simulink model "ctrl_joy"  (R2020b)
settings: Solver=FixedStepAuto  StartTime=0.0  StopTime=Inf  FixedStep=0.01  RelTol=1e-3  EnableMultiTasking=on
model workspace (MAT data in the model file):
  SL_ROS_VariableLengthArrays_MaxSizes.CommonInfo.ArrayTruncateAction = 'EmitWarning'
  SL_ROS_VariableLengthArrays_MaxSizes.MsgTypeMap = containers.Map
  SL_ROS_VariableLengthArrays_MaxSizes.MsgTypeMap.serialization.keys = {'std_msgs/MultiArrayDimension', 'std_msgs/MultiArrayLayout'}
  SL_ROS_VariableLengthArrays_MaxSizes.MsgTypeMap.serialization.values{1}.PropertyName = 'Label'
  SL_ROS_VariableLengthArrays_MaxSizes.MsgTypeMap.serialization.values{1}.DataType = 'uint8'
  SL_ROS_VariableLengthArrays_MaxSizes.MsgTypeMap.serialization.values{1}.MaxLength = 2
  SL_ROS_VariableLengthArrays_MaxSizes.MsgTypeMap.serialization.values{2}.PropertyName = 'Dim'
  SL_ROS_VariableLengthArrays_MaxSizes.MsgTypeMap.serialization.values{2}.DataType = 'std_msgs/MultiArrayDimension'
  SL_ROS_VariableLengthArrays_MaxSizes.MsgTypeMap.serialization.values{2}.MaxLength = 1
  SL_ROS_VariableLengthArrays_MaxSizes.MsgTypeMap.serialization.uniformity = 0
  SL_ROS_VariableLengthArrays_MaxSizes.MsgTypeMap.serialization.keyType = 'char'
  SL_ROS_VariableLengthArrays_MaxSizes.MsgTypeMap.serialization.valueType = 'any'
undefined symbols (not defined in the file): Data, Data_SL_Info, Layout
libraries: robotlib x8
settings Model: SimulationMode=external  ExtModeEnableFloating=off  Creator=erlendbasso  LastModifiedBy=erlendbasso
settings SolverCC: PositivePriorityOrder=on
settings OptimizationCC: EnhancedBackFolding=on  PassReuseOutputArgsAs=Individual arguments  ZeroExternalMemoryAtStartup=off  ZeroInternalMemoryAtStartup=off  MaxStackSize=64  OptimizeBlockOrder=speed  DifferentSizesBufferReuse=on  OptimizationCustomize=off  EfficientTunableParamExpr=on
settings DebuggingCC: ParameterTunabilityLossMsg=error
settings HardwareCC: ProdBitPerPointer=32  ProdBitPerSizeT=32  ProdBitPerPtrDiffT=32  ProdLargestAtomicInteger=Long  ProdLargestAtomicFloat=Double  ProdWordSize=32  ProdHWDeviceType=ARM Compatible->ARM Cortex
settings RTWCC: Description=Embedded Coder  SystemTargetFile=ert.tlc  HardwareBoard=Raspberry Pi - Robot Operating System (ROS)  TLCOptions="-aInlineSetEventsForThisBaseRateFcn=TLC_FALSE -aSuppressMultiTaskScheduler=TLC_FALSE  -aRateBasedStepFcn=0"  TemplateMakefile=ert_default_tmf  Toolchain=Catkin  BuildConfiguration=Faster Runs  TargetLang=C++
settings CodeAppCC: ForceParamTrailComments=on  IgnoreCustomStorageClasses=off  OperatorAnnotations=on  SimulinkDataObjDesc=on  SFDataObjDesc=on  InsertBlockDesc=on
settings ERTTargetCC: SupportContinuousTime=on  SupportVariableSizeSignals=on  ExtModeTransport=2  ExtModeMexFile=ext_xcp  ExtModeIntrfLevel=Level2 - Open

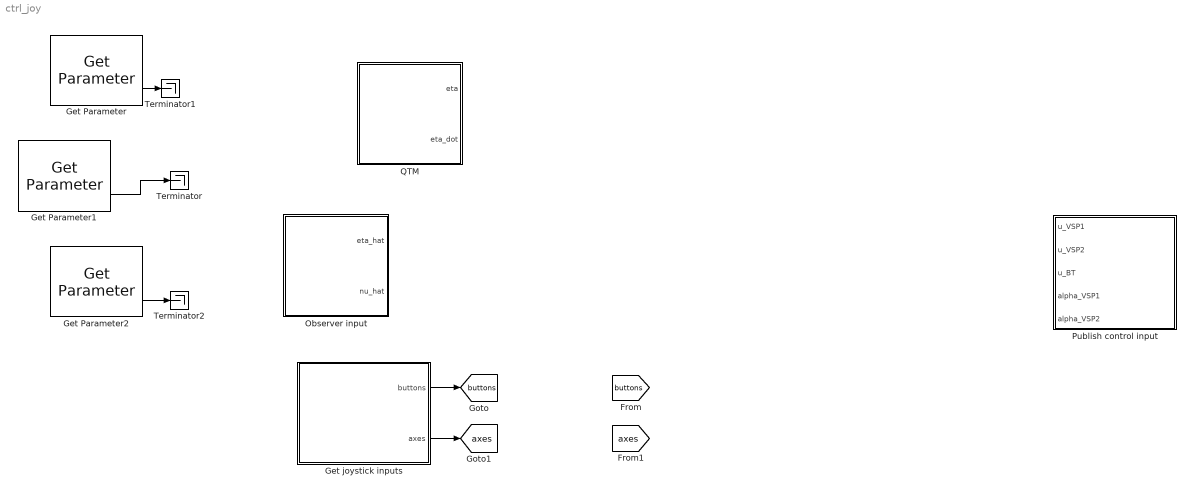
== system ctrl_joy ==
  Get Parameter : robotlib/Get Parameter  ParameterSource=Specify your own  ParameterName=/CSEI/ref/x  ParameterType=double  ParameterMaxArrayLength=16  ParameterInitialValue=0.0  SampleTime=-1  ShowErrorCodeOutput=on  ModelName=ctrl_joy  BlockId=ParamGet_ctrl_joy_537
      settings: SourceProductBaseCode=RR
  Get Parameter1 : robotlib/Get Parameter  ParameterSource=Specify your own  ParameterName=/CSEI/ref/y  ParameterType=double  ParameterMaxArrayLength=16  ParameterInitialValue=0.0  SampleTime=-1  ShowErrorCodeOutput=on  ModelName=ctrl_joy  BlockId=ParamGet_ctrl_joy_539
      settings: SourceProductBaseCode=RR
  Get Parameter2 : robotlib/Get Parameter  ParameterSource=Specify your own  ParameterName=/CSEI/ref/psi  ParameterType=double  ParameterMaxArrayLength=16  ParameterInitialValue=0.0  SampleTime=-1  ShowErrorCodeOutput=on  ModelName=ctrl_joy  BlockId=ParamGet_ctrl_joy_540
      settings: SourceProductBaseCode=RR
  Get joystick inputs : Subsystem
  Observer input : Subsystem
  Publish control input : Subsystem
  QTM : Subsystem
  Terminator : Terminator
  Terminator1 : Terminator
  Terminator2 : Terminator
  tag scope: axes=global, buttons=global
  wires:
  Get joystick inputs/1(buttons) -> [buttons]
  Get joystick inputs/2(axes) -> [axes]
  Get Parameter1/2 -> Terminator/1
  Get Parameter/2 -> Terminator1/1
  Get Parameter2/2 -> Terminator2/1

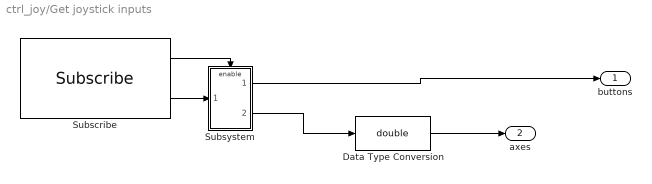
== system ctrl_joy/Get joystick inputs ==
  Data Type Conversion : DataTypeConversion  OutDataTypeStr=double
  Subscribe : robotlib/Subscribe  topicSource=Select from ROS network  topic=/joy  messageType=sensor_msgs/Joy  SampleTime=0.01  legacyBusStruct=off  messageQueueLength=1
  Subsystem : Subsystem
  buttons : Outport
  axes : Outport  Port=2
  wires:
  Subscribe/1 -> Subsystem/Enable
  Subscribe/2 -> Subsystem/1(In1)
  Subsystem/2(<Axes>) -> Data Type Conversion/1
  Subsystem/1(<Buttons>) -> buttons/1
  Data Type Conversion/1 -> axes/1

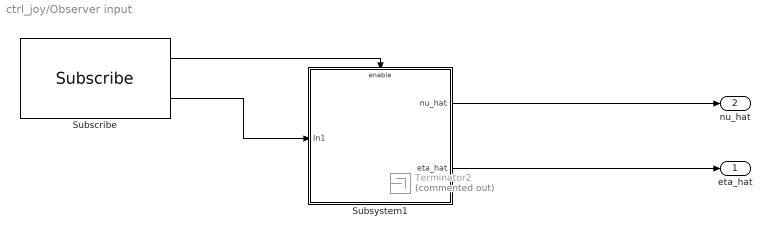
== system ctrl_joy/Observer input ==
  Subscribe : robotlib/Subscribe  topicSource=Specify your own  topic=/observer/odom  messageType=nav_msgs/Odometry  SampleTime=0.01  legacyBusStruct=off  messageQueueLength=1
  Subsystem1 : Subsystem
  Terminator2 : Terminator  Commented=on
  eta_hat : Outport
  nu_hat : Outport  Port=2
  wires:
  Subscribe/2 -> Subsystem1/1(In1)
  Subscribe/1 -> Subsystem1/Enable
  Subsystem1/1(nu_hat) -> nu_hat/1
  Subsystem1/2(eta_hat) -> eta_hat/1

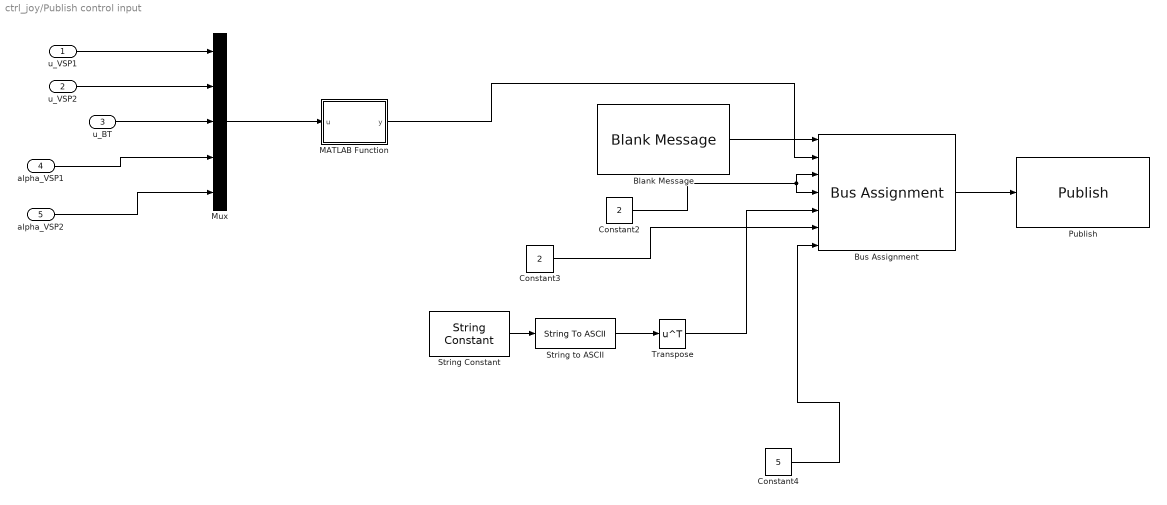
== system ctrl_joy/Publish control input ==
  u_VSP1 : Inport
  u_VSP2 : Inport  Port=2
  u_BT : Inport  Port=3
  alpha_VSP1 : Inport  Port=4
  alpha_VSP2 : Inport  Port=5
  Blank Message : robotlib/Blank Message  messageClass=Message  entityType=std_msgs/Float64MultiArray  messageType=std_msgs/Float64MultiArray  SampleTime=0.01  legacyBusStruct=off
  Bus Assignment : BusAssignment  AssignedSignals=Data,Layout.Dim.Stride,Layout.Dim.Size,Layout.Dim.Label,Layout.Dim.Label_SL_Info.CurrentLength,Data_SL_Info.CurrentLength
  Constant2 : Constant  Value=2  OutDataTypeStr=uint32  SampleTime=Inf
  Constant3 : Constant  Value=2  OutDataTypeStr=uint32  SampleTime=Inf
  Constant4 : Constant  Value=5  OutDataTypeStr=uint32  SampleTime=Inf
  MATLAB Function : MATLAB Function  TreatAsAtomicUnit=on
  Mux : Mux  Inputs=5
  Publish : robotlib/Publish  topicSource=Specify your own  topic=/CSEI/u  messageType=std_msgs/Float64MultiArray  legacyBusStruct=off  messageQueueLength=1
  String Constant : StringConstant  String="\"\""
  String to ASCII : StringToASCII  OutputVectorSize=2
  Transpose : Math  Operator=transpose  SaturateOnIntegerOverflow=on
  wires:
  String Constant/1 -> String to ASCII/1
  Transpose/1 -> Bus Assignment/5
  Bus Assignment/1 -> Publish/1
  Constant3/1 -> Bus Assignment/6
  Constant2/1 -> Bus Assignment/3, Bus Assignment/4
  String to ASCII/1 -> Transpose/1
  Constant4/1 -> Bus Assignment/7
  Blank Message/1 -> Bus Assignment/1
  MATLAB Function/1(y) -> Bus Assignment/2
  alpha_VSP2/1 -> Mux/5
  Mux/1 -> MATLAB Function/1(u)
  alpha_VSP1/1 -> Mux/4
  u_BT/1 -> Mux/3
  u_VSP1/1 -> Mux/1
  u_VSP2/1 -> Mux/2

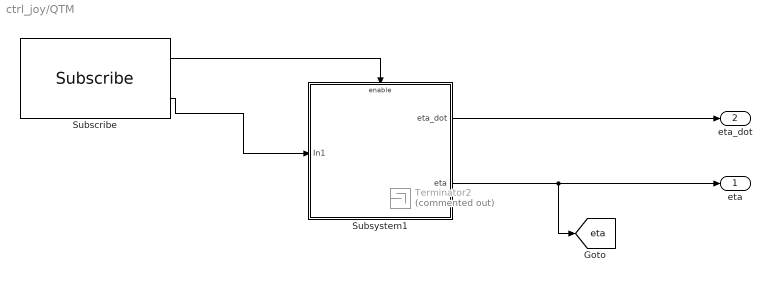
== system ctrl_joy/QTM ==
  Subscribe : robotlib/Subscribe  topicSource=Specify your own  topic=/qualisys/CSEI/odom  messageType=nav_msgs/Odometry  SampleTime=0.01  legacyBusStruct=off  messageQueueLength=1
  Subsystem1 : Subsystem
  Terminator2 : Terminator  Commented=on
  eta : Outport
  eta_dot : Outport  Port=2
  tag scope: eta=global
  wires:
  Subscribe/2 -> Subsystem1/1(In1)
  Subscribe/1 -> Subsystem1/Enable
  Subsystem1/1(eta_dot) -> eta_dot/1
  Subsystem1/2(eta) -> [eta], eta/1

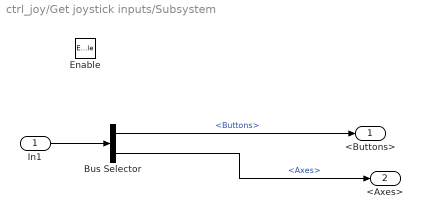
== system ctrl_joy/Get joystick inputs/Subsystem ==
  In1 : Inport
  Enable : EnablePort
  Bus Selector : BusSelector  OutputSignals=Buttons,Axes
  <Buttons> : Outport
  <Axes> : Outport  Port=2
  wires:
  In1/1 -> Bus Selector/1
  Bus Selector/1 -> <Buttons>/1  "<Buttons>"
  Bus Selector/2 -> <Axes>/1  "<Axes>"

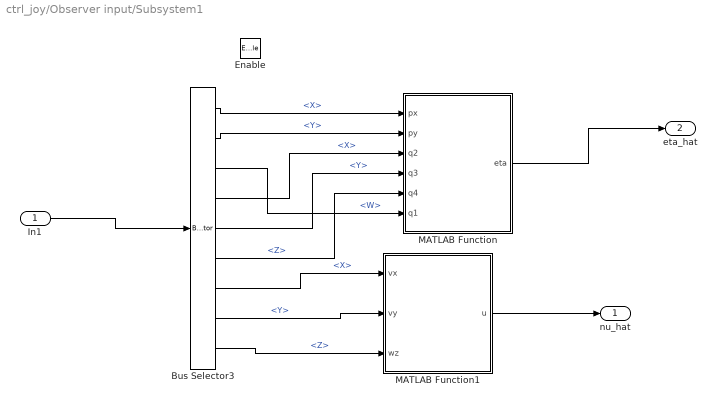
== system ctrl_joy/Observer input/Subsystem1 ==
  In1 : Inport
  Enable : EnablePort
  Bus Selector3 : BusSelector  OutputSignals=Pose.Pose.Position.X,Pose.Pose.Position.Y,Pose.Pose.Orientation.W,Pose.Pose.Orientation.X,Pose.Pose.Orientation.Y,Pose.Pose.Orientation.Z,Twist.Twist.Linear.X,Twist.Twist.Linear.Y,Twist.Twist.Angular.Z
  MATLAB Function : MATLAB Function  TreatAsAtomicUnit=on
  MATLAB Function1 : MATLAB Function  TreatAsAtomicUnit=on
  nu_hat : Outport
  eta_hat : Outport  Port=2
  wires:
  In1/1 -> Bus Selector3/1
  MATLAB Function1/1(u) -> nu_hat/1
  Bus Selector3/7 -> MATLAB Function1/1(vx)  "<X>"
  Bus Selector3/8 -> MATLAB Function1/2(vy)  "<Y>"
  Bus Selector3/9 -> MATLAB Function1/3(wz)  "<Z>"
  MATLAB Function/1(eta) -> eta_hat/1
  Bus Selector3/1 -> MATLAB Function/1(px)  "<X>"
  Bus Selector3/2 -> MATLAB Function/2(py)  "<Y>"
  Bus Selector3/3 -> MATLAB Function/6(q1)  "<W>"
  Bus Selector3/4 -> MATLAB Function/3(q2)  "<X>"
  Bus Selector3/5 -> MATLAB Function/4(q3)  "<Y>"
  Bus Selector3/6 -> MATLAB Function/5(q4)  "<Z>"

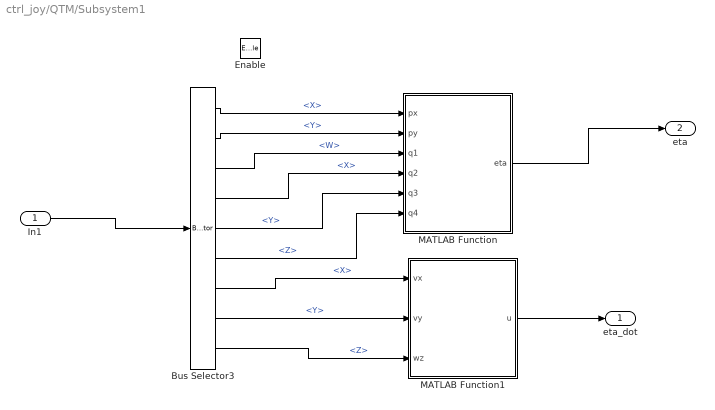
== system ctrl_joy/QTM/Subsystem1 ==
  In1 : Inport
  Enable : EnablePort
  Bus Selector3 : BusSelector  OutputSignals=Pose.Pose.Position.X,Pose.Pose.Position.Y,Pose.Pose.Orientation.W,Pose.Pose.Orientation.X,Pose.Pose.Orientation.Y,Pose.Pose.Orientation.Z,Twist.Twist.Linear.X,Twist.Twist.Linear.Y,Twist.Twist.Angular.Z
  MATLAB Function : MATLAB Function  TreatAsAtomicUnit=on
  MATLAB Function1 : MATLAB Function  TreatAsAtomicUnit=on
  eta_dot : Outport
  eta : Outport  Port=2
  wires:
  In1/1 -> Bus Selector3/1
  MATLAB Function1/1(u) -> eta_dot/1
  MATLAB Function/1(eta) -> eta/1
  Bus Selector3/1 -> MATLAB Function/1(px)  "<X>"
  Bus Selector3/2 -> MATLAB Function/2(py)  "<Y>"
  Bus Selector3/3 -> MATLAB Function/3(q1)  "<W>"
  Bus Selector3/4 -> MATLAB Function/4(q2)  "<X>"
  Bus Selector3/5 -> MATLAB Function/5(q3)  "<Y>"
  Bus Selector3/6 -> MATLAB Function/6(q4)  "<Z>"
  Bus Selector3/9 -> MATLAB Function1/3(wz)  "<Z>"
  Bus Selector3/7 -> MATLAB Function1/1(vx)  "<X>"
  Bus Selector3/8 -> MATLAB Function1/2(vy)  "<Y>"

== matlab function ctrl_joy/Observer input/Subsystem1/MATLAB Function ==
  data: px input; eta output; py input; q2 input; q3 input; q4 input; q1 input
function eta = fcn(px,py,q2,q3,q4,q1)

quat = [q1;q2;q3;q4];
eul = quat2eul(quat','XYZ');

eta = [px;py;eul(3)];

== matlab function ctrl_joy/Observer input/Subsystem1/MATLAB Function1 ==
  data: vx input; u output; vy input; wz input
function u = fcn(vx,vy,wz)

u = [vx;vy;wz];

== matlab function ctrl_joy/Publish control input/MATLAB Function ==
  data: u input; y output
function y = fcn(u)
y = zeros(128,1);

y(1:size(u,1)) = u;

== matlab function ctrl_joy/QTM/Subsystem1/MATLAB Function1 ==
  data: vx input; u output; vy input; wz input
function u = fcn(vx,vy,wz)

u = [vx;vy;wz];

== matlab function ctrl_joy/QTM/Subsystem1/MATLAB Function ==
  data: px input; eta output; py input; q1 input; q2 input; q3 input; q4 input
function eta = fcn(px,py,q1,q2,q3,q4)

quat = [q1;q2;q3;q4];
eul = quat2eul(quat','XYZ');

eta = [px;py;eul(3)];
